simulink model "Speedgoat_V3"  (R2023b)
settings: Solver=FixedStepDiscrete  StartTime=0.0  StopTime=inf  FixedStep=0.001  RelTol=1e-3  EnableMultiTasking=on
model workspace (MAT data in the model file):
  Test = 10000000
undefined symbols (not defined in the file): IO397
libraries: speedgoatlib_fpga_dio x2, simulink x1, simulink_extras x1, speedgoatlib_fpga_analog_io x1, speedgoatlib_fpga x1
(part 2 of 2)

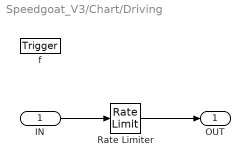
== system Speedgoat_V3/Chart/Driving ==
  IN : Inport  OutMin=[1]  OutMax=[4]  OutDataTypeStr=double  PortDimensions=1
  f : TriggerPort  TriggerType=function-call  VariantControl=(inherit)  SampleTimeType=periodic  SampleTime=0.001
      settings: CopyFcn=Stateflow.SLINSF.SimulinkMan.removeBlockPreDeleteFcn  PreDeleteFcn=Stateflow.SLINSF.SimulinkMan.unsafePredeleteFcn
  Rate Limiter : RateLimiter  RisingSlewLimit=0.01  FallingSlewLimit=-0.01  SampleTimeMode=inherited  InitialCondition=1
  OUT : Outport  OutMin=[1]  OutMax=[4]  OutputWhenDisabled=reset  InitialOutput=[1]
  wires:
  Rate Limiter/1 -> OUT/1
  IN/1 -> Rate Limiter/1

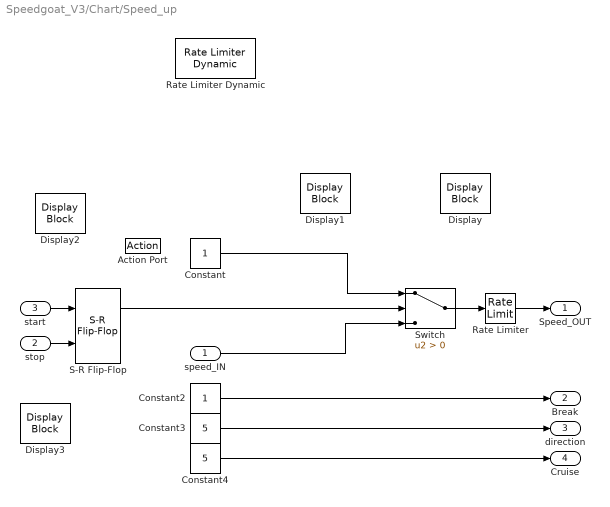
== system Speedgoat_V3/Chart/Speed_up ==
  speed_IN : Inport
  stop : Inport  Port=2  OutMin=[0]  OutMax=[1]
  start : Inport  Port=3  OutMin=[0]  OutMax=[1]
  Action Port : ActionPort
      settings: CopyFcn=Stateflow.SLINSF.SimulinkMan.removeBlockPreDeleteFcn  PreDeleteFcn=Stateflow.SLINSF.SimulinkMan.unsafePredeleteFcn
  Constant : Constant
  Constant2 : Constant
  Constant3 : Constant  Value=5
  Constant4 : Constant  Value=5
  Display{,1..3} (4 alike) : DisplayBlock  LabelPosition=Hide  Transparency=1
  Rate Limiter : RateLimiter  RisingSlewLimit=0.001  FallingSlewLimit=-0.001  SampleTimeMode=inherited  InitialCondition=1
  Rate Limiter Dynamic : simulink/Discontinuities/Rate Limiter Dynamic
  S-R Flip-Flop : simulink_extras/Flip Flops/S-R Flip-Flop  initial_condition=0
  Switch : Switch  Criteria=u2 > Threshold  SaturateOnIntegerOverflow=off  InputSameDT=off
  Speed_OUT : Outport
  Break : Outport  Port=2
  direction : Outport  Port=3
  Cruise : Outport  Port=4
  wires:
  S-R Flip-Flop/1 -> Switch/2
  Constant/1 -> Switch/1
  speed_IN/1 -> Switch/3
  Constant3/1 -> direction/1
  Constant2/1 -> Break/1
  Constant4/1 -> Cruise/1
  start/1 -> S-R Flip-Flop/1
  stop/1 -> S-R Flip-Flop/2
  Rate Limiter/1 -> Speed_OUT/1
  Switch/1 -> Rate Limiter/1

== stateflow chart Speedgoat_V3/Chart ==
  state OUT = Driving(IN) [function]
  state Distance
    du: Speed_OUT = distance_IN;
    du: Driving(distance_IN);
    du: Break = 1;
    du: direction = 5;
    du: Cruise = 5;
  state IDLE
    du: Speed_OUT = 1;
    du: Driving(1);
    du: Break = 5;
    du: direction = 5;
    du: Cruise = 5;
  state Drive
    du: Speed_OUT = Driving(speed_IN);
    du: Break = 1;
    du: direction = 5;
    du: Cruise = 5;
  state Speed_up
  state Stop
    du: Speed_OUT = Driving(1);
    du: Break = 1;
    du: direction = 5;
    du: Cruise = 5;
  Distance -> IDLE [order 2] : [[Emergency_stop == 1]]
  Distance -> IDLE [order 1] : [Speed_OUT == 1]
  (default) -> IDLE
  Drive -> IDLE [order 1] : [[Emergency_stop == 1]]
  IDLE -> Drive : [start == 1]
  Drive -> Distance [order 3] : [distance_IN < 3.5]
  Drive -> Stop [order 2] : [stop == 1]
  Stop -> IDLE : [Speed_OUT == 1]
  Distance -> Stop [order 3] : [stop == 1]
  data: IN function_input double size=1; OUT function_output; sf_internal_action_state_placeholder_data local double size=1 =0; Speed_OUT output; speed_IN input; distance_IN input; start input; stop input; Break output; Emergency_stop input; direction output; Cruise output
